simulink model "AAI"  (R2022a)
settings: Solver=FixedStepAuto  StartTime=0.0  StopTime=10.0  FixedStep=1e-3  RelTol=1e-3  EnableMultiTasking=on
undefined symbols (not defined in the file): D0, D10, D11, D12, D13, D2, D3, D4, D5, D6, D7, D8, D9, PTA0, PTA1, PTA2, PTB23, PTB9, PTC16, PTC2, PTC3, PTC4, PTD0, PTD1, PTD2, PTD3
libraries: frdmk64flib x14
settings Model: ExtModeTrigDuration=5  Creator=12791  LastModifiedBy=simll
settings OptimizationCC: EnhancedBackFolding=on  PassReuseOutputArgsAs=Individual arguments  ZeroExternalMemoryAtStartup=off  ZeroInternalMemoryAtStartup=off  MaxStackSize=64  OptimizeBlockOrder=speed  DifferentSizesBufferReuse=on  OptimizationCustomize=off  EfficientTunableParamExpr=on
settings DebuggingCC: ParameterTunabilityLossMsg=error
settings HardwareCC: ProdBitPerPointer=32  ProdBitPerSizeT=32  ProdBitPerPtrDiffT=32  ProdLargestAtomicInteger=Long  ProdLargestAtomicFloat=Double  ProdWordSize=32  ProdHWDeviceType=ARM Compatible->ARM Cortex
settings SFSimCC: MATLABDynamicMemAlloc=off
settings RTWCC: SystemTargetFile=ert.tlc  HardwareBoard=NXP FRDM-K64F  TLCOptions="-aInlineSetEventsForThisBaseRateFcn=TLC_FALSE -aSuppressMultiTaskScheduler=TLC_FALSE  -aRateBasedStepFcn=0"  TemplateMakefile=ert_default_tmf  Toolchain=GNU Tools for ARM Embedded Processors
settings CodeAppCC: ForceParamTrailComments=on  IgnoreCustomStorageClasses=off  OperatorAnnotations=on  SimulinkDataObjDesc=on  SFDataObjDesc=on  InsertBlockDesc=on
settings ERTTargetCC: ExtModeTransport=4  ExtModeMexFile=sendToCommService

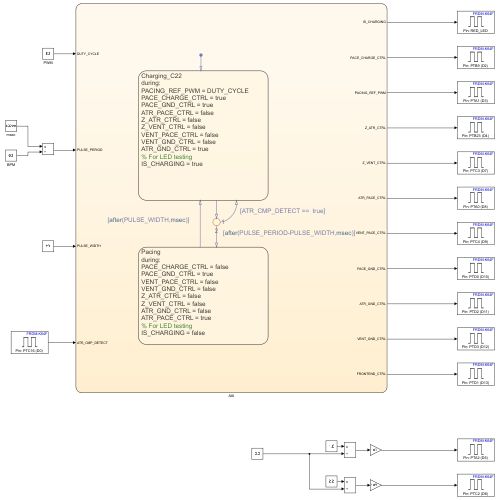
[thumbnail: Simulink's stored preview of the top-level diagram]
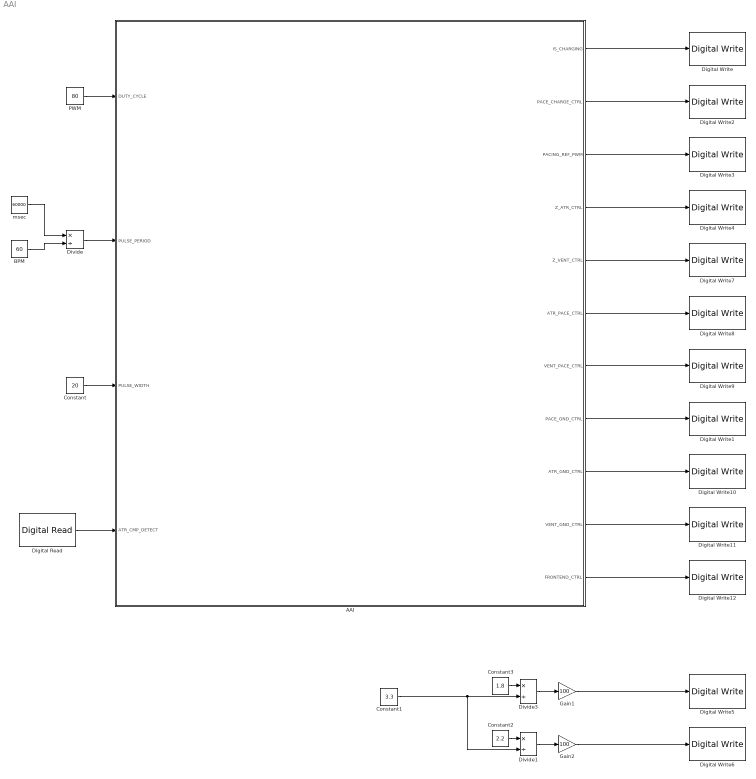
== system AAI ==
  AAI : Stateflow chart  TreatAsAtomicUnit=on
  BPM : Constant  Value=60
  Constant : Constant  Value=20
  Constant1 : Constant  Value=3.3
  Constant2 : Constant  Value=2.2
  Constant3 : Constant  Value=1.8
  Digital Read : frdmk64flib/Digital Read  Whichpin=PTC16 (D0)  SampleTime=-1
  Digital Write : frdmk64flib/Digital Write  Whichpin=RED_LED
  Digital Write1 : frdmk64flib/Digital Write  Whichpin=PTD0 (D10)
  Digital Write10 : frdmk64flib/Digital Write  Whichpin=PTD2 (D11)
  Digital Write11 : frdmk64flib/Digital Write  Whichpin=PTD3 (D12)
  Digital Write12 : frdmk64flib/Digital Write  Whichpin=PTD1 (D13)
  Digital Write2 : frdmk64flib/Digital Write  Whichpin=PTB9 (D2)
  Digital Write3 : frdmk64flib/Digital Write  Whichpin=PTA1 (D3)
  Digital Write4 : frdmk64flib/Digital Write  Whichpin=PTB23 (D4)
  Digital Write5 : frdmk64flib/Digital Write  Whichpin=PTA2 (D5)
  Digital Write6 : frdmk64flib/Digital Write  Whichpin=PTC2 (D6)
  Digital Write7 : frdmk64flib/Digital Write  Whichpin=PTC3 (D7)
  Digital Write8 : frdmk64flib/Digital Write  Whichpin=PTA0 (D8)
  Digital Write9 : frdmk64flib/Digital Write  Whichpin=PTC4 (D9)
  Divide : Product  Inputs=*/
  Divide1 : Product  Inputs=*/
  Divide3 : Product  Inputs=*/
  Gain1 : Gain  Gain=100
  Gain2 : Gain  Gain=100
  PWM : Constant  Value=80
  msec : Constant  Value=60000
  wires:
  AAI/2(PACE_CHARGE_CTRL) -> Digital Write2/1
  AAI/3(PACING_REF_PWM) -> Digital Write3/1
  AAI/4(Z_ATR_CTRL) -> Digital Write4/1
  AAI/5(Z_VENT_CTRL) -> Digital Write7/1
  AAI/6(ATR_PACE_CTRL) -> Digital Write8/1
  AAI/7(VENT_PACE_CTRL) -> Digital Write9/1
  AAI/8(PACE_GND_CTRL) -> Digital Write1/1
  AAI/9(ATR_GND_CTRL) -> Digital Write10/1
  AAI/10(VENT_GND_CTRL) -> Digital Write11/1
  AAI/11(FRONTEND_CTRL) -> Digital Write12/1
  PWM/1 -> AAI/1(DUTY_CYCLE)
  Constant/1 -> AAI/3(PULSE_WIDTH)
  Divide/1 -> AAI/2(PULSE_PERIOD)
  msec/1 -> Divide/1
  BPM/1 -> Divide/2
  AAI/1(IS_CHARGING) -> Digital Write/1
  Divide3/1 -> Gain1/1
  Divide1/1 -> Gain2/1
  Constant1/1 -> Divide3/2, Divide1/2
  Gain1/1 -> Digital Write5/1
  Gain2/1 -> Digital Write6/1
  Constant3/1 -> Divide3/1
  Constant2/1 -> Divide1/1
  Digital Read/1 -> AAI/4(ATR_CMP_DETECT)

== stateflow chart AAI/AAI ==
  state Charging_C22
    during:
    PACING_REF_PWM = DUTY_CYCLE
    PACE_CHARGE_CTRL = true
    PACE_GND_CTRL = true
    ATR_PACE_CTRL = false
    Z_ATR_CTRL = false
    Z_VENT_CTRL = false
    VENT_PACE_CTRL = false
    VENT_GND_CTRL = false
    ATR_GND_CTRL = true
    % For LED testing
    IS_CHARGING = true
  state Pacing
    during:
    PACE_CHARGE_CTRL = false
    PACE_GND_CTRL = true
    VENT_PACE_CTRL = false
    VENT_GND_CTRL = false
    Z_ATR_CTRL = false
    Z_VENT_CTRL = false
    ATR_GND_CTRL = false
    ATR_PACE_CTRL = true
    % For LED testing
    IS_CHARGING = false
  (default) -> Charging_C22
  Pacing -> Charging_C22 : [after(PULSE_WIDTH,msec)]
  Charging_C22 -> (junction 40)
  (junction 40) -> Charging_C22 [order 1] : [ATR_CMP_DETECT ==  true]
  (junction 40) -> Pacing [order 2] : [after(PULSE_PERIOD-PULSE_WIDTH,msec)]
  data: IS_CHARGING output; PACE_CHARGE_CTRL output; PACING_REF_PWM output; Z_ATR_CTRL output; Z_VENT_CTRL output; ATR_PACE_CTRL output; VENT_PACE_CTRL output; PACE_GND_CTRL output; ATR_GND_CTRL output; VENT_GND_CTRL output; FRONTEND_CTRL output =true; DUTY_CYCLE input; PULSE_PERIOD input; PULSE_WIDTH input; ATR_CMP_DETECT input
